simulink library "adjustable_check_valve_v0"  (R2024b)
settings: Solver=VariableStepAuto  StartTime=0.0  StopTime=10.0  RelTol=1e-3
undefined symbols (not defined in the file): ACV_disk_radius, ACV_expansion_factor, ACV_inlet_length, ACV_throat_length
libraries: simulink x2
settings Model: Creator=cmmcguir  LastModifiedBy=cmmcguir

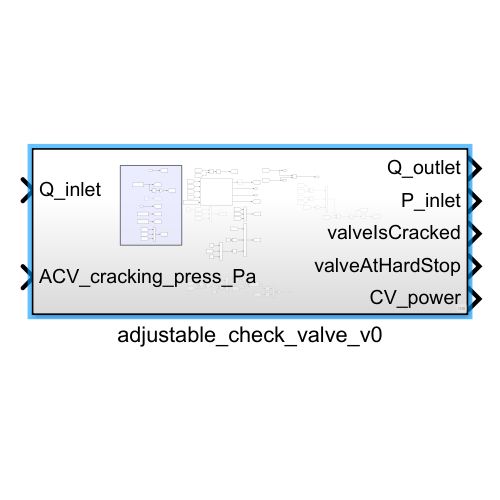
[thumbnail: Simulink's stored preview of the top-level diagram]
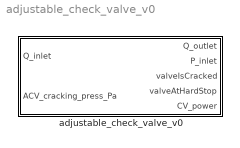
== system adjustable_check_valve_v0 ==
  adjustable_check_valve_v0 : Subsystem

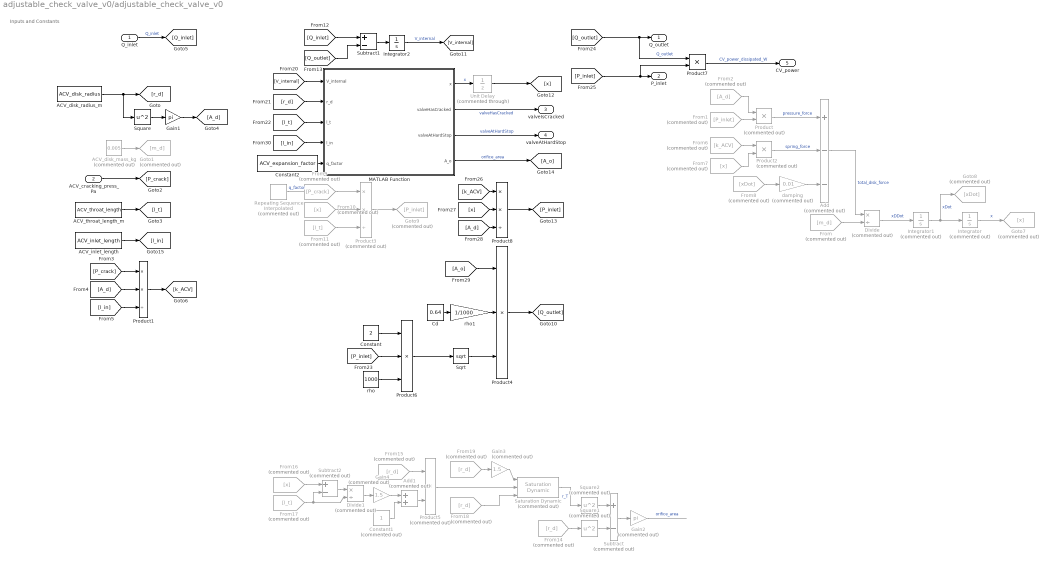
== system adjustable_check_valve_v0/adjustable_check_valve_v0 ==
  note: Inputs and Constants
  Q_inlet : Inport
  ACV_cracking_press_Pa : Inport  Port=2
  ACV_disk_mass_kg : Constant  Commented=on  Value=0.005
  ACV_disk_radius_m : Constant  Value=ACV_disk_radius
  ACV_inlet_length : Constant  Value=ACV_inlet_length
  ACV_throat_length_m : Constant  Value=ACV_throat_length
  Add : Sum  Commented=on  Inputs=+--
  Add1 : Sum  Commented=on
  Cd : Constant  Value=0.64
  Constant : Constant  Value=2
  Constant1 : Constant  Commented=on
  Constant2 : Constant  Value=ACV_expansion_factor
  Divide : Product  Commented=on  Inputs=*/
  Divide1 : Product  Commented=on  Inputs=*/
  From : From  Commented=on  GotoTag=m_d
  From1 : From  Commented=on  GotoTag=P_inlet
  From10 : From  Commented=on  GotoTag=x
  From11 : From  Commented=on  GotoTag=l_t
  From{14..15,18..19} (4 alike) : From  Commented=on  GotoTag=r_d
  From16 : From  Commented=on  GotoTag=x
  From17 : From  Commented=on  GotoTag=l_t
  From2 : From  Commented=on  GotoTag=A_d
  From6 : From  Commented=on  GotoTag=k_ACV
  From7 : From  Commented=on  GotoTag=x
  From8 : From  Commented=on  GotoTag=xDot
  From9 : From  Commented=on  GotoTag=P_crack
  Gain1 : Gain  Gain=pi
  Gain2 : Gain  Commented=on  Gain=pi
  Gain3 : Gain  Commented=on  Gain=1.5
  Gain4 : Gain  Commented=on  Gain=1.5
  Goto1 : Goto  Commented=on  GotoTag=m_d
  Goto7 : Goto  Commented=on  GotoTag=x
  Goto8 : Goto  Commented=on  GotoTag=xDot
  Goto9 : Goto  Commented=on  GotoTag=P_inlet
  Integrator : Integrator  Commented=on
  Integrator1 : Integrator  Commented=on
  Integrator2 : Integrator  InitialCondition=1e-6
  MATLAB Function : MATLAB Function  TreatAsAtomicUnit=on
  Product : Product  Commented=on
  Product1 : Product  Inputs=**/
  Product2 : Product  Commented=on
  Product3 : Product  Commented=on  Inputs=**/
  Product4 : Product  Inputs=***
  Product5 : Product  Commented=on  Inputs=**
  Product6 : Product  Inputs=***
  Product7 : Product
  Product8 : Product  Inputs=**/
  Repeating Sequence Interpolated : simulink/Sources/Repeating Sequence Interpolated  Commented=on  OutValues=[1.01 1.2 1.01]  TimeValues=[0 60 120] * 4  LookUpMeth=Interpolation-Use End Values  tsamp=simu.dt  OutMin=[]  OutMax=[]  OutDataTypeStr=double  OutputDataTypeScalingMode=double  OutDataType=fixdt(0,8)  OutScaling=2^-10
  Saturation Dynamic : simulink/Discontinuities/Saturation Dynamic  Commented=on  OutMin=[]  OutMax=[]  OutDataTypeStr=Inherit: Same as second input  OutDataType=fixdt(1, 16)  OutScaling=2^-10  DoSatur=off
  Sqrt : Sqrt
  Square : Math  Operator=square
  Square1 : Math  Commented=on  Operator=square
  Square2 : Math  Commented=on  Operator=square
  Subtract : Sum  Commented=on  Inputs=+-
  Subtract1 : Sum  Inputs=+-
  Subtract2 : Sum  Commented=on  Inputs=+-
  Unit Delay : UnitDelay  Commented=through  SampleTime=-1  HasFrameUpgradeWarning=on
  damping : Gain  Commented=on  Gain=0.01
  rho : Constant  Value=1000
  rho1 : Gain  Gain=1/1000
  Q_outlet : Outport
  P_inlet : Outport  Port=2
  valveIsCracked : Outport  Port=3
  valveAtHardStop : Outport  Port=4
  CV_power : Outport  Port=5
  wires:
  Integrator/1 -> Goto7/1  "x"
  Integrator1/1 -> Goto8/1, Integrator/1  "xDot"
  Divide/1 -> Integrator1/1  "xDDot"
  ACV_disk_radius_m/1 -> Square/1, [r_d]
  ACV_disk_mass_kg/1 -> Goto1/1
  ACV_cracking_press_Pa/1 -> [P_crack]
  ACV_throat_length_m/1 -> [l_t]
  Square/1 -> Gain1/1
  Gain1/1 -> [A_d]
  Q_inlet/1 -> [Q_inlet]  "Q_inlet"
  From/1 -> Divide/2
  Add/1 -> Divide/1  "total_disk_force"
  From1/1 -> Product/2
  Product/1 -> Add/1  "pressure_force"
  From2/1 -> Product/1
  [P_crack] -> Product1/1
  [A_d] -> Product1/2
  [l_in] -> Product1/3
  Product1/1 -> [k_ACV]
  Product2/1 -> Add/2  "spring_force"
  From6/1 -> Product2/1
  From7/1 -> Product2/2
  From8/1 -> damping/1
  damping/1 -> Add/3
  Product3/1 -> Goto9/1
  From9/1 -> Product3/1
  From10/1 -> Product3/2
  From11/1 -> Product3/3
  Product4/1 -> [Q_outlet]
  Subtract/1 -> Gain2/1
  Gain2/1 -> ?  "orifice_area"
  Square1/1 -> Subtract/2
  From14/1 -> Square1/1
  Product5/1 -> Saturation Dynamic/2
  From15/1 -> Product5/1
  From18/1 -> Saturation Dynamic/3
  From19/1 -> Gain3/1
  Gain3/1 -> Saturation Dynamic/1
  Saturation Dynamic/1 -> Square2/1  "r_T"
  Square2/1 -> Subtract/1
  Integrator2/1 -> [V_internal]  "V_internal"
  MATLAB Function/1(x) -> Unit Delay/1  "x"
  [V_internal] -> MATLAB Function/1(V_internal)
  [r_d] -> MATLAB Function/2(r_d)
  [l_t] -> MATLAB Function/3(l_t)
  Cd/1 -> rho1/1
  Sqrt/1 -> Product4/3
  Product6/1 -> Sqrt/1
  Constant/1 -> Product6/1
  [P_inlet] -> Product6/2
  rho/1 -> Product6/3
  [Q_outlet] -> Product7/1, Q_outlet/1  "Q_outlet"
  [P_inlet] -> Product7/2, P_inlet/1
  MATLAB Function/2(valveHasCracked) -> valveIsCracked/1  "valveHasCracked"
  From16/1 -> Subtract2/1
  From17/1 -> Divide1/2, Subtract2/2
  Subtract2/1 -> Divide1/1
  Divide1/1 -> Gain4/1
  Gain4/1 -> Add1/1
  Add1/1 -> Product5/2
  Constant1/1 -> Add1/2
  Product7/1 -> CV_power/1  "CV_power_dissipated_W"
  rho1/1 -> Product4/2
  Product8/1 -> [P_inlet]
  [k_ACV] -> Product8/1
  [x] -> Product8/2
  [A_d] -> Product8/3
  Unit Delay/1 -> [x]
  MATLAB Function/4(A_o) -> [A_o]  "orifice_area"
  [A_o] -> Product4/1
  [Q_inlet] -> Subtract1/1
  [Q_outlet] -> Subtract1/2
  Subtract1/1 -> Integrator2/1
  MATLAB Function/3(valveAtHardStop) -> valveAtHardStop/1  "valveAtHardStop"
  ACV_inlet_length/1 -> [l_in]
  [l_in] -> MATLAB Function/4(l_in)
  Repeating Sequence Interpolated/1 -> ?  "q_factor"
  Constant2/1 -> MATLAB Function/5(q_factor)

== matlab function adjustable_check_valve_v0/MATLAB Function ==
  data: V_internal input; x output; r_d input; l_t input; valveHasCracked output; valveAtHardStop output; A_o output; l_in input; q_factor input
function [x, valveHasCracked, valveAtHardStop, A_o] = calc_disk_displacement(V_internal, r_d, l_t, l_in, q_factor)

x = V_internal / (pi * r_d^2);
valveHasCracked = 0;
valveAtHardStop = 0;
%q = 1.02; % factor between valve housing radius and disk radius
q = q_factor;
r_outer = q*r_d;
A_o = 0; % orifice area

if V_internal <= 1e-8 % valve has reached retraction hard stop
    valveAtHardStop = 1;
    x = 0;
else
    if x > l_in % passed cracking threshold, in expansion region, revise x estimate due to throat expansion
        valveHasCracked = 1;
        V_rem = V_internal - pi * r_d^2 * l_in; % remaining volume
        
        %sym x_frustum
        %eq1 = V_rem == pi * x_frustum / 12 * r_d^2 * (1 + x/l_t + x^2/l_t^2); % volume of frustum
        %x_rem = eval(solve(eq1));
    
        %x_frustum = roots([1, 3*l_t, 3*l_t^2, -3*l_t^2*V_rem/pi/r_d^2]);
        %x_frustum = roots([1, 6*l_t, 12*l_t^2, -12*l_t^2*V_rem/pi/r_d^2]);
        x_frustum = roots([(q-1)^2 / l_t^2, 3*(q-1) / l_t, 3, -3*V_rem/pi/r_d^2]);
        x_rem = x_frustum(imag(x_frustum) == 0); % remove values with imag components
        x_rem = real(x_rem); % enforce real part (coder throws error otherwise)
        x_rem = min(x_rem(x_rem >= 0)); % select smallest positive value in case multiple real solutions are found
        x = l_in + x_rem;
    
        r_outer_exp = interp1([0 l_t], [r_d r_outer], x_rem);
        A_o = pi*(r_outer_exp^2 - r_d^2);
    end
    
    if x > l_in + l_t % past expansion region
        valveHasCracked = 1;
        
        d = r_d;
        b = r_outer;
        V_frustum = pi*l_t/3 * (d^2 + b*d + b^2);
        V_rem = V_internal - pi*r_d^2*l_in - V_frustum;
        x = l_in + l_t + V_rem / (pi*r_outer^2);
    
        A_o = pi*(r_outer^2 - r_d^2);
    end
end
